simulink model "pendulum_simplePID"  (R2024a)
settings: Solver=VariableStepAuto  StartTime=0.0  StopTime=2  RelTol=1e-3
values from neighbouring files (symbols this model uses):
  b1 = 0.3    [main.m]
  b2 = 0    [main.m]
  g = 9.8    [main.m]
  I = (m*l^2) / 3    (= 0.0416666666667)    [main.m]
  l = 0.5    [main.m]
  m = 0.5    [main.m]
  M = 1    [main.m]
  theta0 = 30 * pi/180    (= 0.523598775598)    [main.m]
  theta_d = 0 * pi/180    (= 0)    [main.m]
settings Model: Creator=yiming  LastModifiedBy=yiming

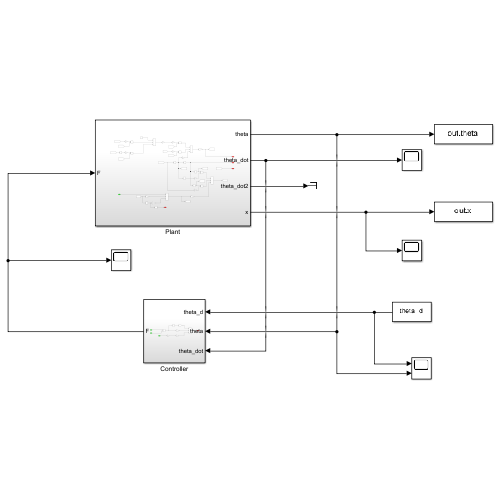
[thumbnail: Simulink's stored preview of the top-level diagram]
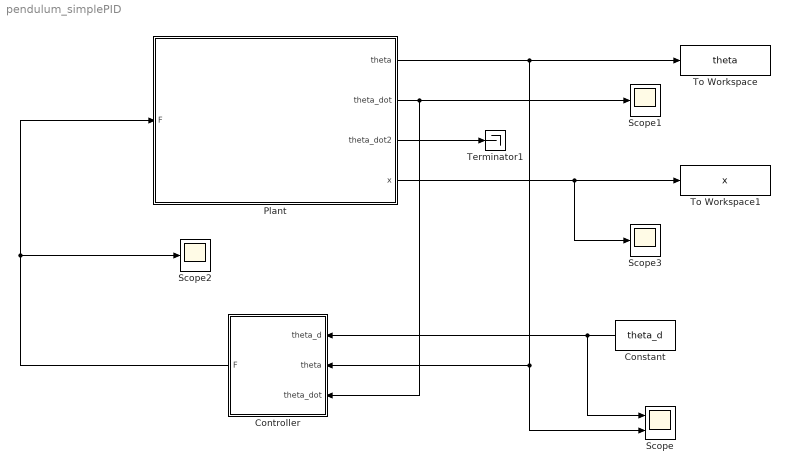
== system pendulum_simplePID ==
  Constant : Constant  Value=theta_d
  Controller : Subsystem
  Plant : Subsystem
  Scope : Scope  NumInputPorts=2
  Scope1 : Scope
  Scope2 : Scope
  Scope3 : Scope
  Terminator1 : Terminator
  To Workspace : ToWorkspace  VariableName=theta  SaveFormat=Timeseries  SampleTime=-1
  To Workspace1 : ToWorkspace  VariableName=x  SaveFormat=Timeseries  SampleTime=-1
  wires:
  Plant/1(theta) -> To Workspace/1, Controller/2(theta), Scope/2
  Plant/3(theta_dot2) -> Terminator1/1
  Constant/1 -> Controller/1(theta_d), Scope/1
  Controller/1(F) -> Scope2/1, Plant/1(F)
  Plant/2(theta_dot) -> Controller/3(theta_dot), Scope1/1
  Plant/4(x) -> Scope3/1, To Workspace1/1

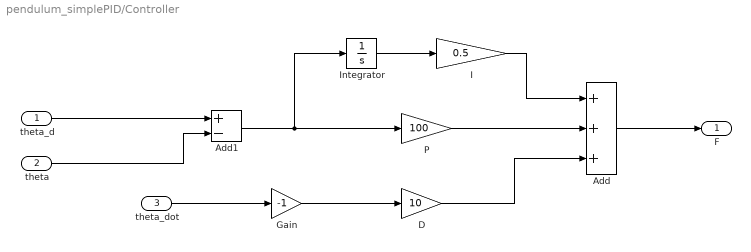
== system pendulum_simplePID/Controller ==
  theta_d : Inport
  theta : Inport  Port=2
  theta_dot : Inport  Port=3
  Add : Sum  Inputs=+++
  Add1 : Sum  Inputs=+-
  D : Gain  Gain=10
  Gain : Gain  Gain=-1
  I : Gain  Gain=0.5
  Integrator : Integrator
  P : Gain  Gain=100
  F : Outport
  wires:
  Integrator/1 -> I/1
  P/1 -> Add/2
  I/1 -> Add/1
  D/1 -> Add/3
  Add/1 -> F/1
  theta_dot/1 -> Gain/1
  Add1/1 -> Integrator/1, P/1
  theta/1 -> Add1/2
  theta_d/1 -> Add1/1
  Gain/1 -> D/1

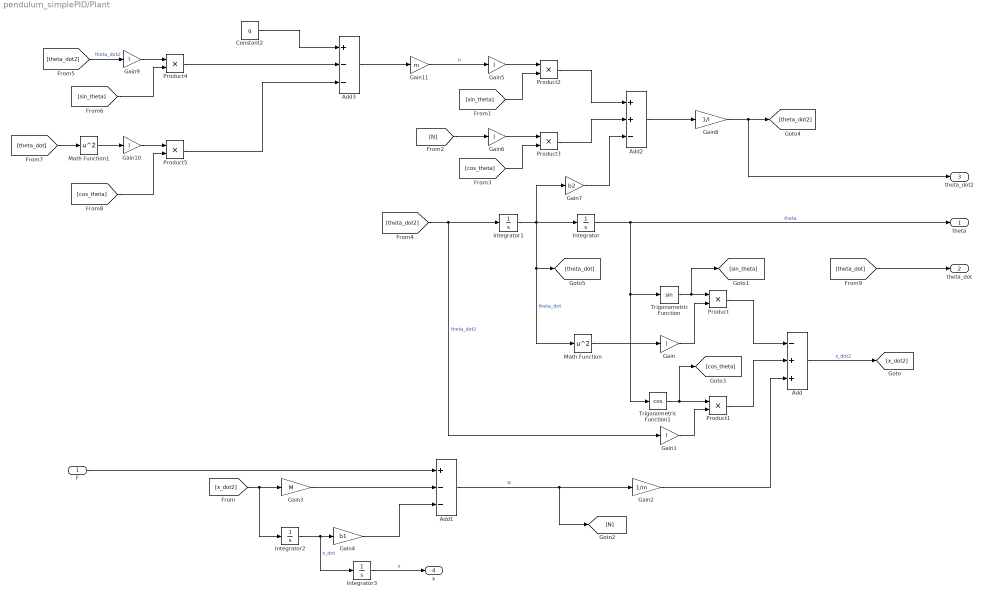
== system pendulum_simplePID/Plant ==
  F : Inport
  Add : Sum  Inputs=-++
  Add1 : Sum  Inputs=+--
  Add2 : Sum  Inputs=++-
  Add3 : Sum  Inputs=+--
  Constant2 : Constant  Value=g
  Gain{,1,5..6,9..10} (6 alike) : Gain  Gain=l
  Gain11 : Gain  Gain=m
  Gain2 : Gain  Gain=1/m
  Gain3 : Gain  Gain=M
  Gain4 : Gain  Gain=b1
  Gain7 : Gain  Gain=b2
  Gain8 : Gain  Gain=1/I
  Integrator : Integrator  InitialCondition=theta0
  Integrator1 : Integrator
  Integrator2 : Integrator
  Integrator3 : Integrator
  Math Function : Math  Operator=square
  Math Function1 : Math  Operator=square
  Product{,1..5} (6 alike) : Product
  Trigonometric Function : Trigonometry
  Trigonometric Function1 : Trigonometry  Operator=cos
  theta : Outport
  theta_dot : Outport  Port=2
  theta_dot2 : Outport  Port=3
  x : Outport  Port=4
  wires:
  Integrator/1 -> theta/1, Trigonometric Function1/1, Trigonometric Function/1  "theta"
  Integrator1/1 -> Gain7/1, Integrator/1, [theta_dot], Math Function/1  "theta_dot"
  Math Function/1 -> Gain/1
  Trigonometric Function/1 -> [sin_theta], Product/1
  Gain/1 -> Product/2
  [theta_dot2] -> Gain1/1, Integrator1/1  "theta_dot2"
  Trigonometric Function1/1 -> Product1/1, [cos_theta]
  Gain1/1 -> Product1/2
  Product1/1 -> Add/2
  Product/1 -> Add/1
  Add1/1 -> [N], Gain2/1  "N"
  Add/1 -> [x_dot2]  "x_dot2"
  Gain2/1 -> Add/3
  [x_dot2] -> Integrator2/1, Gain3/1
  F/1 -> Add1/1
  Gain3/1 -> Add1/2
  Integrator2/1 -> Integrator3/1, Gain4/1  "x_dot"
  Gain4/1 -> Add1/3
  Gain11/1 -> Gain5/1  "P"
  Gain5/1 -> Product2/1
  [sin_theta] -> Product2/2
  [N] -> Gain6/1
  Gain6/1 -> Product3/1
  [cos_theta] -> Product3/2
  Product2/1 -> Add2/1
  Product3/1 -> Add2/2
  Gain7/1 -> Add2/3
  Add2/1 -> Gain8/1
  Gain8/1 -> theta_dot2/1, [theta_dot2]
  [theta_dot2] -> Gain9/1  "theta_dot2"
  Gain9/1 -> Product4/1
  [sin_theta] -> Product4/2
  [theta_dot] -> Math Function1/1
  Math Function1/1 -> Gain10/1
  Gain10/1 -> Product5/1
  [cos_theta] -> Product5/2
  Product4/1 -> Add3/2
  Product5/1 -> Add3/3
  Constant2/1 -> Add3/1
  Add3/1 -> Gain11/1
  [theta_dot] -> theta_dot/1
  Integrator3/1 -> x/1  "x"
